simulink model "Single Phase to Ground Fault"  (R2023a)
settings: Solver=ode3  StartTime=0.0  StopTime=1  FixedStep=Ts  RelTol=1e-4  EnableMultiTasking=on
undefined symbols (not defined in the file): Ts
libraries: spsMeanLib x13, spsabctodq0Lib x12, slpidlib x8, spsThreePhaseSeriesRLCBranchLib x7, spsThreePhaseVIMeasurementLib x7, spsSeriesRLCBranchLib x6, spsPower3phInstantaneousLib x5, spspowerguiLib x3, spsPWMGenerator2LevelLib x2, spsdq0toabcLib x2, spsGroundLib x2, spsUniversalBridgeLib x2
(part 1 of 2)
settings Model: Creator=RAVINDRA  LastModifiedBy=LENOVO
settings SolverCC: AlgebraicLoopSolver=TrustRegion
settings DataIOCC: LimitDataPoints=on  SaveFormat=Array  ReturnWorkspaceOutputs=off
settings OptimizationCC: LifeSpan=inf
settings DebuggingCC: SolverPrmCheckMsg=warning  UnconnectedInputMsg=warning  UnconnectedOutputMsg=warning  UnconnectedLineMsg=warning  SFUnexpectedBacktrackingDiag=warning  SFNoUnconditionalDefaultTransitionDiag=warning  SFExecutionAtInitializationDiag=none  ArithmeticOperatorsInVariantConditions=warning
settings HardwareCC: ProdBitPerPointer=32  ProdBitPerSizeT=32  ProdBitPerPtrDiffT=32  ProdLargestAtomicFloat=None  ProdIntDivRoundTo=Undefined  ProdEndianess=Unspecified  ProdWordSize=32  ProdHWDeviceType=32-bit Generic
settings ModelReferenceCC: PropagateSignalLabelsOutOfModel=off
settings SFSimCC: SimUseLocalCustomCode=off  CustomCodeUndefinedFunction=UseInterfaceOnly
settings RTWCC: RTWUseLocalCustomCode=off
settings CodeAppCC: StateflowObjectComments=on
settings GRTTargetCC: TargetLangStandard=C89/C90 (ANSI)
settings ConfigComp: CovMetricSettings=dw  CovSaveCumulativeToWorkspaceVar=on  CovSaveSingleToWorkspaceVar=on  CovExternalEMLEnable=off  CovSFcnEnable=off
settings SimscapeCC: SimscapeNormalizeSystem=off

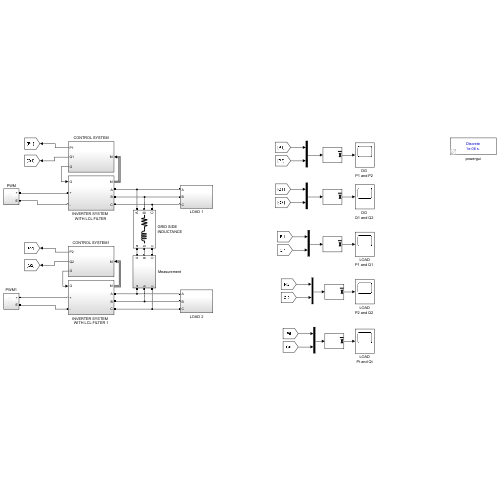
[thumbnail: Simulink's stored preview of the top-level diagram]
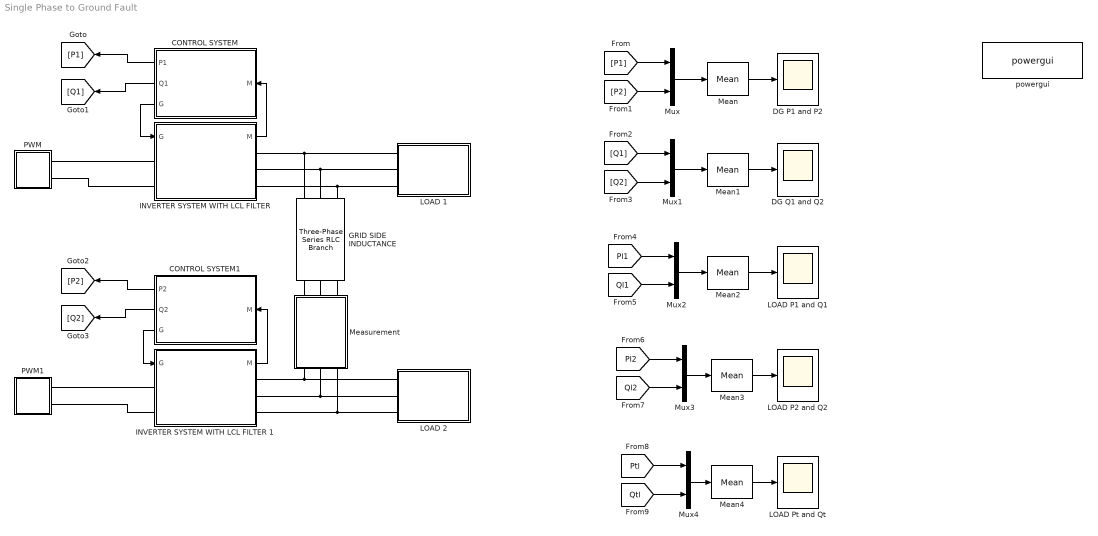
== system Single Phase to Ground Fault ==
  CONTROL SYSTEM : Subsystem
  CONTROL SYSTEM1 : Subsystem
  "DG P1 and P2 " : Scope
  "DG Q1 and Q2 " : Scope
  GRID SIDE INDUCTANCE : spsThreePhaseSeriesRLCBranchLib/Three-Phase Series RLC Branch  LConnTagsString=A|B|C  RConnTagsString=A|B|C  BranchType=RL  Resistance=.55  Inductance=20e-5  Capacitance=1e-6  Measurements=None
  "INVERTER SYSTEM WITH LCL FILTER " : Subsystem
  INVERTER SYSTEM WITH LCL FILTER 1 : Subsystem
  "LOAD P1 and Q1 " : Scope
  "LOAD P2 and Q2 " : Scope
  LOAD Pt and Qt : Scope
  LOAD 1 : Subsystem
  LOAD 2 : Subsystem
  Mean{,1..4} (5 alike) : spsMeanLib/Mean  Freq=60  Vinit=0  Ts=0
  Measurement : Subsystem
  Mux{,1..4} (5 alike) : Mux  Inputs=2
  PWM : Subsystem
  PWM1 : Subsystem
  powergui : spspowerguiLib/powergui  Priority=1  SimulationMode=Discrete  SampleTime=Ts  frequency=60  Iterations=50  frequencyindice=0  Pbase=100e6  ErrMax=1e-4  UnitsV=kV  UnitsW=MW  buscounter=0  FunctionMessages=off  echomessages=off  EnableUseOfTLC=off  CurrentSourceSwitches=off  DisableSnubberDevices=off  DisableRonSwitches=off  DisableVfSwitches=off  DisplayEquations=off  AutomaticDiscreteSolvers=off  SolverType=Tustin  Interpol=off  ExternalGateDelay=off  methode=off  Ts=0  x0status=blocks  SPID=off  SwTol=0  HookPort=off  NonlinearTolerance=1e-4  nMaxIteration=100  ContinueOnMaxIteration=off  RestoreLinks=warning  ResistiveCurrentMeasurement=off  Frange=[0:2:500]  Ylog=off  Xlog=on  ShowGrid=off  save=off  variable=ZData  structure=0  ZoomFFT=off  StartTime=0.0  cycles=1  DisplayStyle=1  fundamental=60  FreqAxis=off  MaxFrequency=1000  frequencyindicesteady=1  RmsSteady=1  display=off
  wires:
  "INVERTER SYSTEM WITH LCL FILTER "/1(M) -> CONTROL SYSTEM/1(M)
  CONTROL SYSTEM/3(G) -> "INVERTER SYSTEM WITH LCL FILTER "/1(G)
  INVERTER SYSTEM WITH LCL FILTER 1/1(M) -> CONTROL SYSTEM1/1(M)
  CONTROL SYSTEM1/3(G) -> INVERTER SYSTEM WITH LCL FILTER 1/1(G)
  CONTROL SYSTEM/1(P1) -> [P1]
  CONTROL SYSTEM/2(Q1) -> [Q1]
  CONTROL SYSTEM1/1(P2) -> [P2]
  CONTROL SYSTEM1/2(Q2) -> [Q2]
  [P1] -> Mux/1
  [P2] -> Mux/2
  Mux/1 -> Mean/1
  [Q1] -> Mux1/1
  [Q2] -> Mux1/2
  [Pl1] -> Mux2/1
  [Ql1] -> Mux2/2
  Mux2/1 -> Mean2/1
  [Pl2] -> Mux3/1
  [Ql2] -> Mux3/2
  [Ptl] -> Mux4/1
  [Qtl] -> Mux4/2
  Mux1/1 -> Mean1/1
  Mux3/1 -> Mean3/1
  Mux4/1 -> Mean4/1
  Mean/1 -> "DG P1 and P2 "/1
  Mean1/1 -> "DG Q1 and Q2 "/1
  Mean2/1 -> "LOAD P1 and Q1 "/1
  Mean3/1 -> "LOAD P2 and Q2 "/1
  Mean4/1 -> LOAD Pt and Qt/1
  connections:
  PWM/LConn1 -- "INVERTER SYSTEM WITH LCL FILTER "/LConn1
  "INVERTER SYSTEM WITH LCL FILTER "/LConn2 -- PWM/LConn2
  LOAD 1/LConn1 -- "INVERTER SYSTEM WITH LCL FILTER "/RConn1 -- GRID SIDE INDUCTANCE/LConn1
  LOAD 1/LConn2 -- "INVERTER SYSTEM WITH LCL FILTER "/RConn2 -- GRID SIDE INDUCTANCE/LConn2
  LOAD 1/LConn3 -- "INVERTER SYSTEM WITH LCL FILTER "/RConn3 -- GRID SIDE INDUCTANCE/LConn3
  INVERTER SYSTEM WITH LCL FILTER 1/RConn1 -- Measurement/LConn1 -- LOAD 2/LConn1
  INVERTER SYSTEM WITH LCL FILTER 1/RConn2 -- Measurement/LConn2 -- LOAD 2/LConn2
  INVERTER SYSTEM WITH LCL FILTER 1/RConn3 -- Measurement/LConn3 -- LOAD 2/LConn3
  INVERTER SYSTEM WITH LCL FILTER 1/LConn1 -- PWM1/LConn1
  PWM1/LConn2 -- INVERTER SYSTEM WITH LCL FILTER 1/LConn2
  Measurement/RConn1 -- GRID SIDE INDUCTANCE/RConn1
  Measurement/RConn2 -- GRID SIDE INDUCTANCE/RConn2
  Measurement/RConn3 -- GRID SIDE INDUCTANCE/RConn3

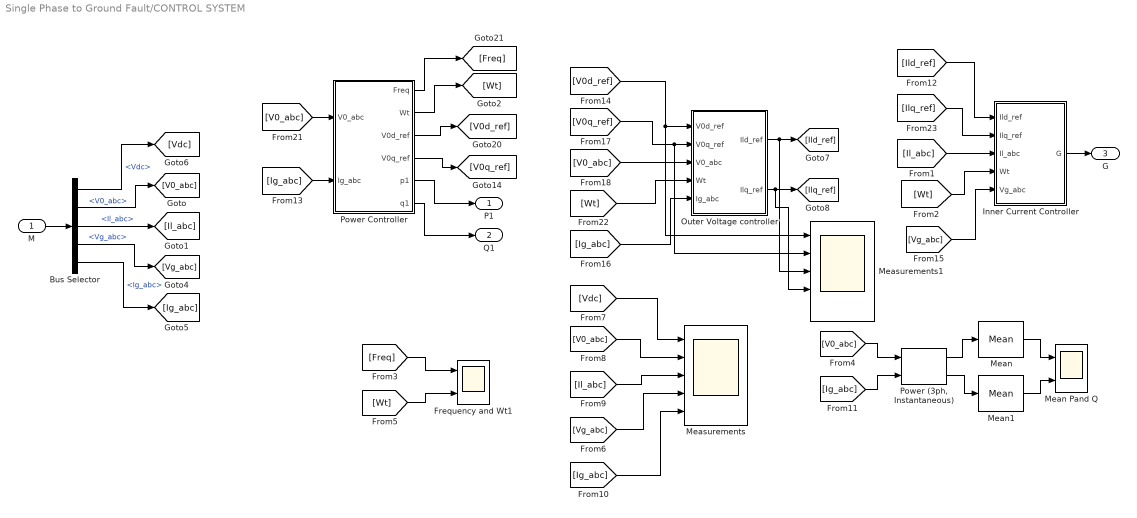
== system Single Phase to Ground Fault/CONTROL SYSTEM ==
  M : Inport
  Bus Selector : BusSelector  OutputSignals=Vdc,V0_abc,Il_abc,Vg_abc,Ig_abc
  Frequency and Wt1 : Scope  NumInputPorts=2
  Inner Current Controller : Subsystem
  Mean : spsMeanLib/Mean  Freq=50  Vinit=0  Ts=0
  Mean Pand Q : Scope  NumInputPorts=2
  Mean1 : spsMeanLib/Mean  Freq=50  Vinit=0  Ts=0
  Measurements : Scope  NumInputPorts=5
  Measurements1 : Scope  NumInputPorts=5
  Outer Voltage controller : Subsystem
  "Power (3ph, Instantaneous)" : spsPower3phInstantaneousLib/Power (3ph, Instantaneous)
  Power Controller : Subsystem
  P1 : Outport
  Q1 : Outport  Port=2
  G : Outport  Port=3
  wires:
  M/1 -> Bus Selector/1
  Bus Selector/1 -> [Vdc]  "<Vdc>"
  Bus Selector/2 -> [V0_abc]  "<V0_abc>"
  Bus Selector/3 -> [Il_abc]  "<Il_abc>"
  Bus Selector/4 -> [Vg_abc]  "<Vg_abc>"
  Bus Selector/5 -> [Ig_abc]  "<Ig_abc>"
  [Vg_abc] -> Measurements/4
  [Vdc] -> Measurements/1
  [V0_abc] -> Measurements/2
  [Il_abc] -> Measurements/3
  [Ig_abc] -> Measurements/5
  [V0_abc] -> Power Controller/1(V0_abc)
  [Ig_abc] -> Power Controller/2(Ig_abc)
  Power Controller/1(Freq) -> [Freq]
  Power Controller/3(V0d_ref) -> [V0d_ref]
  Power Controller/4(V0q_ref) -> [V0q_ref]
  [Wt] -> Frequency and Wt1/2
  Power Controller/2(Wt) -> [Wt]
  [V0d_ref] -> Measurements1/1, Outer Voltage controller/1(V0d_ref)
  [V0q_ref] -> Measurements1/2, Outer Voltage controller/2(V0q_ref)
  [V0_abc] -> Outer Voltage controller/3(V0_abc)
  [Wt] -> Outer Voltage controller/4(Wt)
  Outer Voltage controller/1(Ild_ref) -> Measurements1/3, [Ild_ref]
  Outer Voltage controller/2(Ilq_ref) -> Measurements1/4, [Ilq_ref]
  [Freq] -> Frequency and Wt1/1
  [Ild_ref] -> Inner Current Controller/1(Ild_ref)
  [Ilq_ref] -> Inner Current Controller/2(Ilq_ref)
  [Il_abc] -> Inner Current Controller/3(Il_abc)
  Inner Current Controller/1(G) -> G/1
  [Wt] -> Inner Current Controller/4(Wt)
  [Vg_abc] -> Inner Current Controller/5(Vg_abc)
  [Ig_abc] -> Outer Voltage controller/5(Ig_abc)
  Power Controller/5(p1) -> P1/1
  Power Controller/6(q1) -> Q1/1
  [Ig_abc] -> "Power (3ph, Instantaneous)"/2
  [V0_abc] -> "Power (3ph, Instantaneous)"/1
  "Power (3ph, Instantaneous)"/1 -> Mean/1
  Mean/1 -> Mean Pand Q/1
  Mean1/1 -> Mean Pand Q/2
  "Power (3ph, Instantaneous)"/2 -> Mean1/1

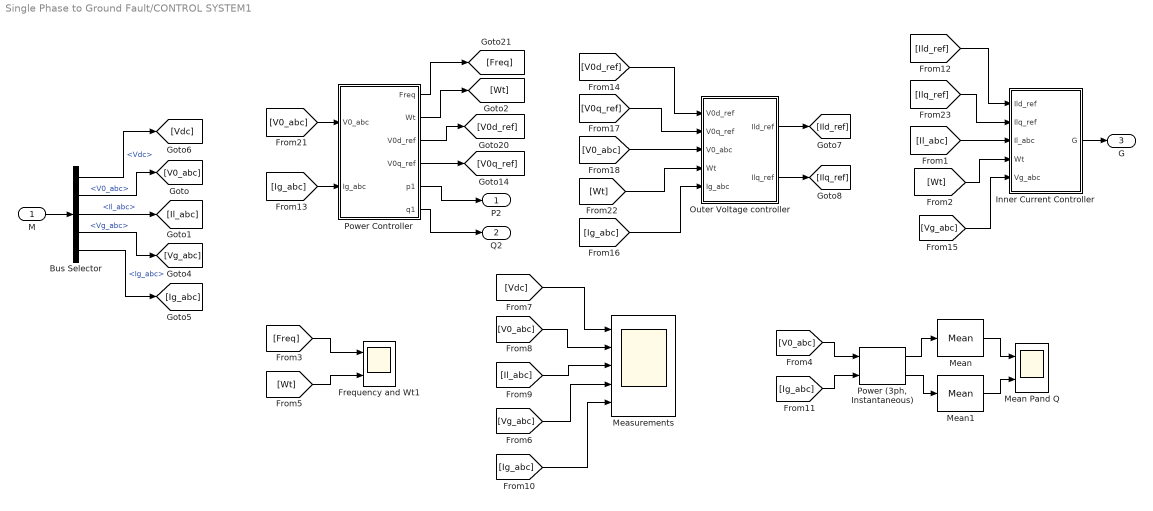
== system Single Phase to Ground Fault/CONTROL SYSTEM1 ==
  M : Inport
  Bus Selector : BusSelector  OutputSignals=Vdc,V0_abc,Il_abc,Vg_abc,Ig_abc
  Frequency and Wt1 : Scope  NumInputPorts=2
  Inner Current Controller : Subsystem
  Mean : spsMeanLib/Mean  Freq=50  Vinit=0  Ts=0
  Mean Pand Q : Scope  NumInputPorts=2
  Mean1 : spsMeanLib/Mean  Freq=50  Vinit=0  Ts=0
  Measurements : Scope  NumInputPorts=5
  Outer Voltage controller : Subsystem
  "Power (3ph, Instantaneous)" : spsPower3phInstantaneousLib/Power (3ph, Instantaneous)
  Power Controller : Subsystem
  P2 : Outport
  Q2 : Outport  Port=2
  G : Outport  Port=3
  wires:
  [Ig_abc] -> Outer Voltage controller/5(Ig_abc)
  [Vg_abc] -> Inner Current Controller/5(Vg_abc)
  [Wt] -> Inner Current Controller/4(Wt)
  Inner Current Controller/1(G) -> G/1
  [Il_abc] -> Inner Current Controller/3(Il_abc)
  [Ilq_ref] -> Inner Current Controller/2(Ilq_ref)
  [Ild_ref] -> Inner Current Controller/1(Ild_ref)
  "Power (3ph, Instantaneous)"/2 -> Mean1/1
  Mean1/1 -> Mean Pand Q/2
  Mean/1 -> Mean Pand Q/1
  "Power (3ph, Instantaneous)"/1 -> Mean/1
  [V0_abc] -> "Power (3ph, Instantaneous)"/1
  [Ig_abc] -> "Power (3ph, Instantaneous)"/2
  [Freq] -> Frequency and Wt1/1
  Outer Voltage controller/2(Ilq_ref) -> [Ilq_ref]
  Outer Voltage controller/1(Ild_ref) -> [Ild_ref]
  [Wt] -> Outer Voltage controller/4(Wt)
  [V0_abc] -> Outer Voltage controller/3(V0_abc)
  [V0q_ref] -> Outer Voltage controller/2(V0q_ref)
  [V0d_ref] -> Outer Voltage controller/1(V0d_ref)
  [Wt] -> Frequency and Wt1/2
  [Ig_abc] -> Measurements/5
  [Il_abc] -> Measurements/3
  [V0_abc] -> Measurements/2
  [Vdc] -> Measurements/1
  [Vg_abc] -> Measurements/4
  Bus Selector/5 -> [Ig_abc]  "<Ig_abc>"
  Bus Selector/4 -> [Vg_abc]  "<Vg_abc>"
  Bus Selector/3 -> [Il_abc]  "<Il_abc>"
  Bus Selector/2 -> [V0_abc]  "<V0_abc>"
  Bus Selector/1 -> [Vdc]  "<Vdc>"
  M/1 -> Bus Selector/1
  [V0_abc] -> Power Controller/1(V0_abc)
  [Ig_abc] -> Power Controller/2(Ig_abc)
  Power Controller/1(Freq) -> [Freq]
  Power Controller/3(V0d_ref) -> [V0d_ref]
  Power Controller/4(V0q_ref) -> [V0q_ref]
  Power Controller/2(Wt) -> [Wt]
  Power Controller/5(p1) -> P2/1
  Power Controller/6(q1) -> Q2/1

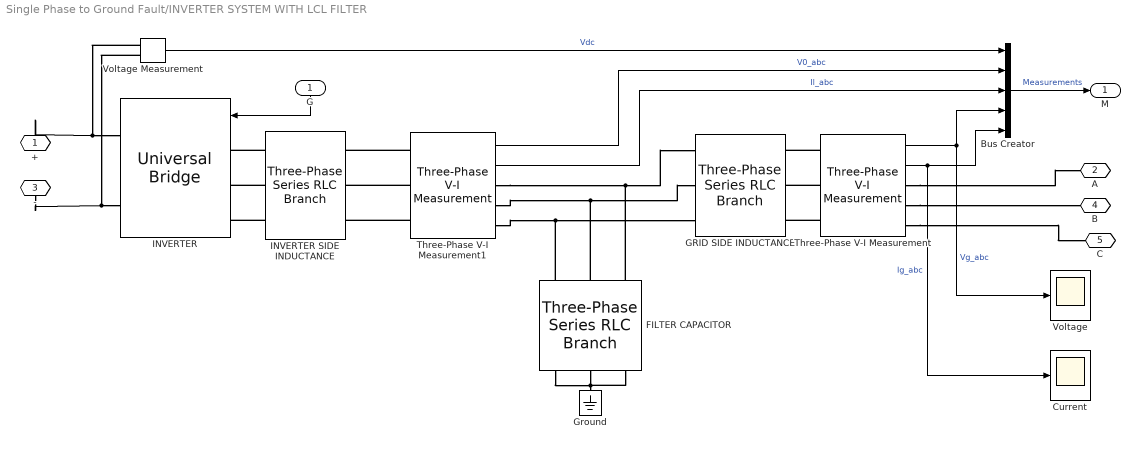
== system Single Phase to Ground Fault/INVERTER SYSTEM WITH LCL FILTER  ==
  G : Inport
  Bus Creator : BusCreator  Inputs=5
  Current : Scope
  FILTER CAPACITOR : spsThreePhaseSeriesRLCBranchLib/Three-Phase Series RLC Branch  LConnTagsString=A|B|C  RConnTagsString=A|B|C  BranchType=RC  Resistance=5  Inductance=1e-3  Capacitance=15e-6  Measurements=None
  GRID SIDE INDUCTANCE : spsThreePhaseSeriesRLCBranchLib/Three-Phase Series RLC Branch  LConnTagsString=A|B|C  RConnTagsString=A|B|C  BranchType=RL  Resistance=0.2  Inductance=1e-3  Capacitance=1e-6  Measurements=None
  Ground : spsGroundLib/Ground  LConnTagsString=a
  INVERTER : spsUniversalBridgeLib/Universal Bridge  Arms=3  SnubberResistance=1e5  SnubberCapacitance=inf  Device=IGBT / Diodes  Ron=1e-3  Lon=0  ForwardVoltages="[  0  0  ]"  ForwardVoltage=0  GTOparameters=[ 10e-6 , 20e-6 ]  IGBTparameters=[ 1e-6 , 2e-6 ]  Measurements=None  Measurements_2=None  converterType=Rectifier
  INVERTER SIDE INDUCTANCE : spsThreePhaseSeriesRLCBranchLib/Three-Phase Series RLC Branch  LConnTagsString=A|B|C  RConnTagsString=A|B|C  BranchType=RL  Resistance=0.2  Inductance=2e-3  Capacitance=1e-6  Measurements=None
  Three-Phase V-I Measurement : spsThreePhaseVIMeasurementLib/Three-Phase V-I Measurement  VoltageMeasurement=phase-to-ground  SetLabelV=off  LabelV=Vabc  Vpu=off  VpuLL=off  CurrentMeasurement=yes  SetLabelI=off  LabelI=Iabc  Ipu=off  Pbase=100e6  Vbase=500e3  OutputType=Complex  PhasorSimulation=off  PSBequivalent=0
  Three-Phase V-I Measurement1 : spsThreePhaseVIMeasurementLib/Three-Phase V-I Measurement  VoltageMeasurement=phase-to-ground  SetLabelV=off  LabelV=V0_abc  Vpu=off  VpuLL=off  CurrentMeasurement=yes  SetLabelI=off  LabelI=Iabc  Ipu=off  Pbase=100e6  Vbase=500e3  OutputType=Complex  PhasorSimulation=off  PSBequivalent=0
  Voltage : Scope
  Voltage Measurement : spsVoltageMeasurementLib/Voltage Measurement  PhasorSimulation=off  OutputType=Complex  PSBequivalent=0
  + : PMIOPort  Side=Left
  A : PMIOPort  Port=2  Side=Right
  - : PMIOPort  Port=3  Side=Left
  B : PMIOPort  Port=4  Side=Right
  C : PMIOPort  Port=5  Side=Right
  M : Outport
  wires:
  Bus Creator/1 -> M/1  "Measurements"
  G/1 -> INVERTER/1
  Three-Phase V-I Measurement/1 -> Voltage/1, Bus Creator/4  "Vg_abc"
  Three-Phase V-I Measurement1/1 -> Bus Creator/2  "V0_abc"
  Three-Phase V-I Measurement1/2 -> Bus Creator/3  "Il_abc"
  Voltage Measurement/1 -> Bus Creator/1  "Vdc"
  Three-Phase V-I Measurement/2 -> Current/1, Bus Creator/5  "Ig_abc"
  connections:
  INVERTER SIDE INDUCTANCE/LConn1 -- INVERTER/LConn1
  Three-Phase V-I Measurement1/LConn1 -- INVERTER SIDE INDUCTANCE/RConn1
  Three-Phase V-I Measurement1/LConn2 -- INVERTER SIDE INDUCTANCE/RConn2
  Voltage Measurement/LConn2 -- -/RConn1 -- INVERTER/RConn2
  Three-Phase V-I Measurement1/LConn3 -- INVERTER SIDE INDUCTANCE/RConn3
  Voltage Measurement/LConn1 -- +/RConn1 -- INVERTER/RConn1
  FILTER CAPACITOR/LConn2 -- GRID SIDE INDUCTANCE/LConn2 -- Three-Phase V-I Measurement1/RConn2
  Three-Phase V-I Measurement/RConn1 -- A/RConn1
  Three-Phase V-I Measurement/RConn3 -- C/RConn1
  INVERTER SIDE INDUCTANCE/LConn3 -- INVERTER/LConn3
  INVERTER SIDE INDUCTANCE/LConn2 -- INVERTER/LConn2
  Three-Phase V-I Measurement/RConn2 -- B/RConn1
  Three-Phase V-I Measurement/LConn1 -- GRID SIDE INDUCTANCE/RConn1
  Three-Phase V-I Measurement/LConn2 -- GRID SIDE INDUCTANCE/RConn2
  FILTER CAPACITOR/LConn1 -- GRID SIDE INDUCTANCE/LConn3 -- Three-Phase V-I Measurement1/RConn3
  FILTER CAPACITOR/RConn1 -- FILTER CAPACITOR/RConn3 -- Ground/LConn1 -- FILTER CAPACITOR/RConn2
  FILTER CAPACITOR/LConn3 -- GRID SIDE INDUCTANCE/LConn1 -- Three-Phase V-I Measurement1/RConn1
  Three-Phase V-I Measurement/LConn3 -- GRID SIDE INDUCTANCE/RConn3

== system Single Phase to Ground Fault/INVERTER SYSTEM WITH LCL FILTER 1 ==
  G : Inport
  Bus Creator : BusCreator  Inputs=5
  FILTER CAPACITOR : spsThreePhaseSeriesRLCBranchLib/Three-Phase Series RLC Branch  LConnTagsString=A|B|C  RConnTagsString=A|B|C  BranchType=RC  Resistance=5  Inductance=1e-3  Capacitance=15e-6  Measurements=None
  GRID SIDE INDUCTANCE : spsThreePhaseSeriesRLCBranchLib/Three-Phase Series RLC Branch  LConnTagsString=A|B|C  RConnTagsString=A|B|C  BranchType=RL  Resistance=0.2  Inductance=1e-3  Capacitance=1e-6  Measurements=None
  Ground : spsGroundLib/Ground  LConnTagsString=a
  INVERTER : spsUniversalBridgeLib/Universal Bridge  Arms=3  SnubberResistance=1e5  SnubberCapacitance=inf  Device=IGBT / Diodes  Ron=1e-3  Lon=0  ForwardVoltages="[  0  0  ]"  ForwardVoltage=0  GTOparameters=[ 10e-6 , 20e-6 ]  IGBTparameters=[ 1e-6 , 2e-6 ]  Measurements=None  Measurements_2=None  converterType=Rectifier
  INVERTER SIDE INDUCTANCE : spsThreePhaseSeriesRLCBranchLib/Three-Phase Series RLC Branch  LConnTagsString=A|B|C  RConnTagsString=A|B|C  BranchType=RL  Resistance=0.2  Inductance=2e-3  Capacitance=1e-6  Measurements=None
  Three-Phase V-I Measurement : spsThreePhaseVIMeasurementLib/Three-Phase V-I Measurement  VoltageMeasurement=phase-to-ground  SetLabelV=off  LabelV=Vabc  Vpu=off  VpuLL=off  CurrentMeasurement=yes  SetLabelI=off  LabelI=Iabc  Ipu=off  Pbase=100e6  Vbase=500e3  OutputType=Complex  PhasorSimulation=off  PSBequivalent=0
  Three-Phase V-I Measurement1 : spsThreePhaseVIMeasurementLib/Three-Phase V-I Measurement  VoltageMeasurement=phase-to-ground  SetLabelV=off  LabelV=V0_abc  Vpu=off  VpuLL=off  CurrentMeasurement=yes  SetLabelI=off  LabelI=Iabc  Ipu=off  Pbase=100e6  Vbase=500e3  OutputType=Complex  PhasorSimulation=off  PSBequivalent=0
  Voltage Measurement : spsVoltageMeasurementLib/Voltage Measurement  PhasorSimulation=off  OutputType=Complex  PSBequivalent=0
  + : PMIOPort  Side=Left
  A : PMIOPort  Port=2  Side=Right
  - : PMIOPort  Port=3  Side=Left
  B : PMIOPort  Port=4  Side=Right
  C : PMIOPort  Port=5  Side=Right
  M : Outport
  wires:
  Three-Phase V-I Measurement/2 -> Bus Creator/5  "Ig_abc"
  Voltage Measurement/1 -> Bus Creator/1  "Vdc"
  Three-Phase V-I Measurement1/2 -> Bus Creator/3  "Il_abc"
  Three-Phase V-I Measurement1/1 -> Bus Creator/2  "V0_abc"
  Three-Phase V-I Measurement/1 -> Bus Creator/4  "Vg_abc"
  G/1 -> INVERTER/1
  Bus Creator/1 -> M/1  "Measurements"
  connections:
  Three-Phase V-I Measurement/LConn3 -- GRID SIDE INDUCTANCE/RConn3
  Three-Phase V-I Measurement1/RConn1 -- GRID SIDE INDUCTANCE/LConn1 -- FILTER CAPACITOR/LConn3
  FILTER CAPACITOR/RConn2 -- Ground/LConn1 -- FILTER CAPACITOR/RConn3 -- FILTER CAPACITOR/RConn1
  Three-Phase V-I Measurement1/RConn3 -- GRID SIDE INDUCTANCE/LConn3 -- FILTER CAPACITOR/LConn1
  Three-Phase V-I Measurement/LConn2 -- GRID SIDE INDUCTANCE/RConn2
  Three-Phase V-I Measurement/LConn1 -- GRID SIDE INDUCTANCE/RConn1
  Three-Phase V-I Measurement/RConn2 -- B/RConn1
  INVERTER SIDE INDUCTANCE/LConn2 -- INVERTER/LConn2
  INVERTER SIDE INDUCTANCE/LConn3 -- INVERTER/LConn3
  Three-Phase V-I Measurement/RConn3 -- C/RConn1
  Three-Phase V-I Measurement/RConn1 -- A/RConn1
  Three-Phase V-I Measurement1/RConn2 -- GRID SIDE INDUCTANCE/LConn2 -- FILTER CAPACITOR/LConn2
  INVERTER/RConn1 -- +/RConn1 -- Voltage Measurement/LConn1
  Three-Phase V-I Measurement1/LConn3 -- INVERTER SIDE INDUCTANCE/RConn3
  INVERTER/RConn2 -- -/RConn1 -- Voltage Measurement/LConn2
  Three-Phase V-I Measurement1/LConn2 -- INVERTER SIDE INDUCTANCE/RConn2
  Three-Phase V-I Measurement1/LConn1 -- INVERTER SIDE INDUCTANCE/RConn1
  INVERTER SIDE INDUCTANCE/LConn1 -- INVERTER/LConn1

== system Single Phase to Ground Fault/LOAD 1 ==
  Mean : spsMeanLib/Mean  Freq=50  Vinit=0  Ts=0
  Mean Pand Q : Scope  NumInputPorts=2
  Mean1 : spsMeanLib/Mean  Freq=50  Vinit=0  Ts=0
  "Power (3ph, Instantaneous)" : spsPower3phInstantaneousLib/Power (3ph, Instantaneous)
  Three-Phase Series RLC Load : spsThreePhaseSeriesRLCLoadLib/Three-Phase Series RLC Load  LConnTagsString=A|B|C  Configuration=Y (grounded)  NominalVoltage=400  Vabc=[1e3 1e3 1e3]  Vabcp=[1e3 1e3 1e3]  NominalFrequency=50  UnbalancedPower=off  ActivePower=7000  InductivePower=0  CapacitivePower=0  Pabc=[10e3 9e3 11e3]  QLabc=[100 90 110]  QCabc=[100 90 110]  Pabcp=[10e3 9e3 11e3]  QLabcp=[100 90 110]  QCabcp=[100 90 110]  Measurements=None  LoadType=constant Z
  Three-Phase V-I Measurement : spsThreePhaseVIMeasurementLib/Three-Phase V-I Measurement  VoltageMeasurement=phase-to-ground  SetLabelV=off  LabelV=Vabc  Vpu=off  VpuLL=off  CurrentMeasurement=yes  SetLabelI=off  LabelI=Iabc  Ipu=off  Pbase=100e6  Vbase=500e3  OutputType=Complex  PhasorSimulation=off  PSBequivalent=0
  Three-Phase Fault : spsThreePhaseFaultLib/Three-Phase Fault  InitialStates=0  FaultA=on  FaultB=off  FaultC=off  GroundFault=on  SwitchTimes=[0.1 0.168]  External=off  SwitchStatus=NaN  FaultResistance=8  GroundResistance=0.01  SnubberResistance=1e6  SnubberCapacitance=inf  Measurements=None
  A : PMIOPort  Side=Left
  B : PMIOPort  Port=2  Side=Left
  C : PMIOPort  Port=3  Side=Left
  tag scope: Pl1=global, Ql1=global
  wires:
  [Il1_abc] -> "Power (3ph, Instantaneous)"/2
  [Vl1_abc] -> "Power (3ph, Instantaneous)"/1
  "Power (3ph, Instantaneous)"/1 -> [Pl1], Mean/1
  Mean/1 -> Mean Pand Q/1
  Mean1/1 -> Mean Pand Q/2
  "Power (3ph, Instantaneous)"/2 -> [Ql1], Mean1/1
  Three-Phase V-I Measurement/2 -> [Il1_abc]
  Three-Phase V-I Measurement/1 -> [Vl1_abc]
  connections:
  Three-Phase V-I Measurement/LConn1 -- Three-Phase Fault/LConn1 -- A/RConn1
  Three-Phase V-I Measurement/LConn2 -- Three-Phase Fault/LConn2 -- B/RConn1
  Three-Phase V-I Measurement/LConn3 -- Three-Phase Fault/LConn3 -- C/RConn1
  Three-Phase V-I Measurement/RConn1 -- Three-Phase Series RLC Load/LConn1
  Three-Phase V-I Measurement/RConn2 -- Three-Phase Series RLC Load/LConn2
  Three-Phase V-I Measurement/RConn3 -- Three-Phase Series RLC Load/LConn3

== system Single Phase to Ground Fault/LOAD 2 ==
  Mean : spsMeanLib/Mean  Freq=50  Vinit=0  Ts=0
  Mean Pand Q : Scope  NumInputPorts=2
  Mean1 : spsMeanLib/Mean  Freq=50  Vinit=0  Ts=0
  "Power (3ph, Instantaneous)" : spsPower3phInstantaneousLib/Power (3ph, Instantaneous)
  Three-Phase Series RLC Load : spsThreePhaseSeriesRLCLoadLib/Three-Phase Series RLC Load  LConnTagsString=A|B|C  Configuration=Y (grounded)  NominalVoltage=400  Vabc=[1e3 1e3 1e3]  Vabcp=[1e3 1e3 1e3]  NominalFrequency=50  UnbalancedPower=off  ActivePower=3000  InductivePower=0  CapacitivePower=0  Pabc=[10e3 9e3 11e3]  QLabc=[100 90 110]  QCabc=[100 90 110]  Pabcp=[10e3 9e3 11e3]  QLabcp=[100 90 110]  QCabcp=[100 90 110]  Measurements=None  LoadType=constant Z
  Three-Phase V-I Measurement : spsThreePhaseVIMeasurementLib/Three-Phase V-I Measurement  VoltageMeasurement=phase-to-ground  SetLabelV=off  LabelV=Vabc  Vpu=off  VpuLL=off  CurrentMeasurement=yes  SetLabelI=off  LabelI=Iabc  Ipu=off  Pbase=100e6  Vbase=500e3  OutputType=Complex  PhasorSimulation=off  PSBequivalent=0
  Three-Phase Fault : spsThreePhaseFaultLib/Three-Phase Fault  InitialStates=0  FaultA=on  FaultB=off  FaultC=off  GroundFault=on  SwitchTimes=[0.1 0.168]  External=off  SwitchStatus=NaN  FaultResistance=8  GroundResistance=0.01  SnubberResistance=1e6  SnubberCapacitance=inf  Measurements=None
  A : PMIOPort  Side=Left
  B : PMIOPort  Port=2  Side=Left
  C : PMIOPort  Port=3  Side=Left
  tag scope: Pl2=global, Ql2=global
  wires:
  [Il2_abc] -> "Power (3ph, Instantaneous)"/2
  [Vl2_abc] -> "Power (3ph, Instantaneous)"/1
  "Power (3ph, Instantaneous)"/1 -> [Pl2], Mean/1
  Mean/1 -> Mean Pand Q/1
  Mean1/1 -> Mean Pand Q/2
  "Power (3ph, Instantaneous)"/2 -> [Ql2], Mean1/1
  Three-Phase V-I Measurement/2 -> [Il2_abc]
  Three-Phase V-I Measurement/1 -> [Vl2_abc]
  connections:
  Three-Phase Series RLC Load/LConn1 -- Three-Phase V-I Measurement/RConn1
  Three-Phase Series RLC Load/LConn3 -- Three-Phase V-I Measurement/RConn3
  Three-Phase Series RLC Load/LConn2 -- Three-Phase V-I Measurement/RConn2
  A/RConn1 -- Three-Phase Fault/LConn1 -- Three-Phase V-I Measurement/LConn1
  B/RConn1 -- Three-Phase Fault/LConn2 -- Three-Phase V-I Measurement/LConn2
  C/RConn1 -- Three-Phase Fault/LConn3 -- Three-Phase V-I Measurement/LConn3

== system Single Phase to Ground Fault/Measurement ==
  "Power (3ph, Instantaneous)" : spsPower3phInstantaneousLib/Power (3ph, Instantaneous)
  Three-Phase V-I Measurement : spsThreePhaseVIMeasurementLib/Three-Phase V-I Measurement  VoltageMeasurement=phase-to-ground  SetLabelV=off  LabelV=Vabc  Vpu=off  VpuLL=off  CurrentMeasurement=yes  SetLabelI=off  LabelI=Iabc  Ipu=off  Pbase=100e6  Vbase=500e3  OutputType=Complex  PhasorSimulation=off  PSBequivalent=0
  A : PMIOPort  Side=Right
  B : PMIOPort  Port=2  Side=Right
  C : PMIOPort  Port=3  Side=Right
  a : PMIOPort  Port=4  Side=Left
  b : PMIOPort  Port=5  Side=Left
  c : PMIOPort  Port=6  Side=Left
  tag scope: Ptl=global, Qtl=global
  wires:
  Three-Phase V-I Measurement/1 -> "Power (3ph, Instantaneous)"/1
  Three-Phase V-I Measurement/2 -> "Power (3ph, Instantaneous)"/2
  "Power (3ph, Instantaneous)"/1 -> [Ptl]
  "Power (3ph, Instantaneous)"/2 -> [Qtl]
  connections:
  A/RConn1 -- Three-Phase V-I Measurement/LConn1
  B/RConn1 -- Three-Phase V-I Measurement/LConn2
  C/RConn1 -- Three-Phase V-I Measurement/LConn3
  a/RConn1 -- Three-Phase V-I Measurement/RConn1
  b/RConn1 -- Three-Phase V-I Measurement/RConn2
  c/RConn1 -- Three-Phase V-I Measurement/RConn3

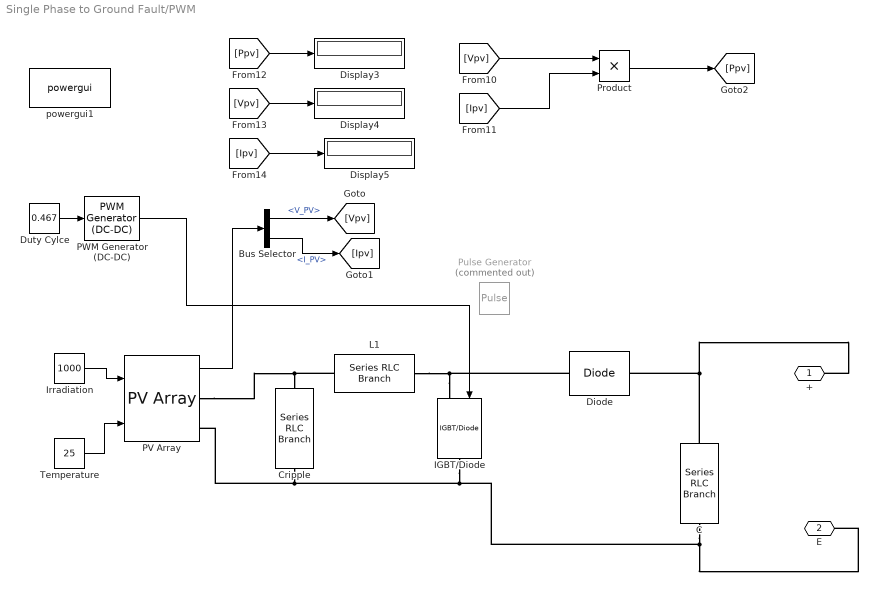
== system Single Phase to Ground Fault/PWM ==
  Bus Selector : BusSelector  OutputSignals=V_PV,I_PV
  C : spsSeriesRLCBranchLib/Series RLC Branch  LConnTagsString=__new0  RConnTagsString=__new0  BranchType=C  Resistance=0  Inductance=0  SetiL0=off  InitialCurrent=0  Capacitance=0.000000207  Setx0=off  InitialVoltage=0  Measurements=None
  Cripple : spsSeriesRLCBranchLib/Series RLC Branch  LConnTagsString=__new0  RConnTagsString=__new0  BranchType=C  Resistance=0  Inductance=0  SetiL0=off  InitialCurrent=0  Capacitance=0.006  Setx0=off  InitialVoltage=0  Measurements=None
  Diode : spsDiodeLib/Diode  Ron=0.001  Lon=0  Vf=0.8  IC=0  UseSnubber=0  Rs=500  Cs=250e-9  Measurements=off
  Display3 : Display
  Display4 : Display
  Display5 : Display
  Duty Cylce : Constant  Value=0.467
  IGBT/Diode : spsIGBTDiodeLib/IGBT//Diode  Ron=1e-3  Rs=1e5  Cs=inf  Measurements=off
  Irradiation : Constant  Value=1000
  L1 : spsSeriesRLCBranchLib/Series RLC Branch  LConnTagsString=__new0  RConnTagsString=__new0  BranchType=L  Resistance=0  Inductance=0.000349  SetiL0=off  InitialCurrent=0  Capacitance=0.006  Setx0=off  InitialVoltage=0  Measurements=None
  PV Array : spsPVArrayLib/PV Array  Npar=5  Nser=10  PlotType=array @ 1000 W/m2 & specified temperatures  S_vec="[ 1000  500  100 ]"  Temp_C_vec="[ 45 25  ]"  ModuleName=User-defined  PlotWhenSelected=off  Pm=200  Ncell=5.8  Voc=41  Isc=6  Vm=40  Im=5  beta_Voc_pc=-0.36099  alpha_Isc_pc=0.102  beta_Voc=-0.14801  alpha_Isc=0.00612  IL=7.0494  I0=8.7017e-23  nI=5.8087  Rsh=8.8608  Rs=0.0024678  RobustModel=off  RobustCellTemperature=25  BAL=on  Tc=1e-6  Tfilter=5e-5
  PWM Generator (DC-DC) : spsPWMGeneratorDCDCLib/PWM Generator (DC-DC)  Fsw=20000  Ts=Ts
  Product : Product
  Pulse Generator : DiscretePulseGenerator  Commented=on  PulseType=Time based  Period=5e-05  PulseWidth=0.002
  Temperature : Constant  Value=25
  powergui1 : spspowerguiLib/powergui  Priority=1  SimulationMode=Discrete  SampleTime=1e-6  frequency=60  Iterations=50  frequencyindice=0  Pbase=100e6  ErrMax=1e-4  UnitsV=kV  UnitsW=MW  buscounter=0  FunctionMessages=off  echomessages=off  EnableUseOfTLC=off  CurrentSourceSwitches=off  DisableSnubberDevices=off  DisableRonSwitches=off  DisableVfSwitches=off  DisplayEquations=off  AutomaticDiscreteSolvers=off  SolverType=Tustin/Backward Euler (TBE)  Interpol=off  ExternalGateDelay=off  methode=off  Ts=100  x0status=blocks  SPID=on  SwTol=0  HookPort=off  NonlinearTolerance=1e-4  nMaxIteration=100  ContinueOnMaxIteration=off  RestoreLinks=warning  ResistiveCurrentMeasurement=off  Frange=[0:2:500]  Ylog=off  Xlog=on  ShowGrid=off  save=off  variable=ZData  structure=0  ZoomFFT=off  StartTime=0.0  cycles=1  DisplayStyle=1  fundamental=60  FreqAxis=off  MaxFrequency=1000  frequencyindicesteady=1  RmsSteady=1  display=off
  + : PMIOPort  Side=Left
  E : PMIOPort  Port=2  Side=Left
  wires:
  [Vpv] -> Display4/1
  Bus Selector/2 -> [Ipv]  "<I_PV>"
  Bus Selector/1 -> [Vpv]  "<V_PV>"
  [Ipv] -> Display5/1
  [Ppv] -> Display3/1
  [Vpv] -> Product/1
  Irradiation/1 -> PV Array/1
  PWM Generator (DC-DC)/1 -> IGBT/Diode/1
  [Ipv] -> Product/2
  Duty Cylce/1 -> PWM Generator (DC-DC)/1
  Product/1 -> [Ppv]
  PV Array/1 -> Bus Selector/1
  Temperature/1 -> PV Array/2
  connections:
  Cripple/LConn1 -- PV Array/RConn1 -- L1/RConn1
  C/LConn1 -- Diode/RConn1 -- +/RConn1
  IGBT/Diode/LConn1 -- L1/LConn1 -- Diode/LConn1
  PV Array/RConn2 -- Cripple/RConn1 -- IGBT/Diode/RConn1 -- C/RConn1 -- E/RConn1

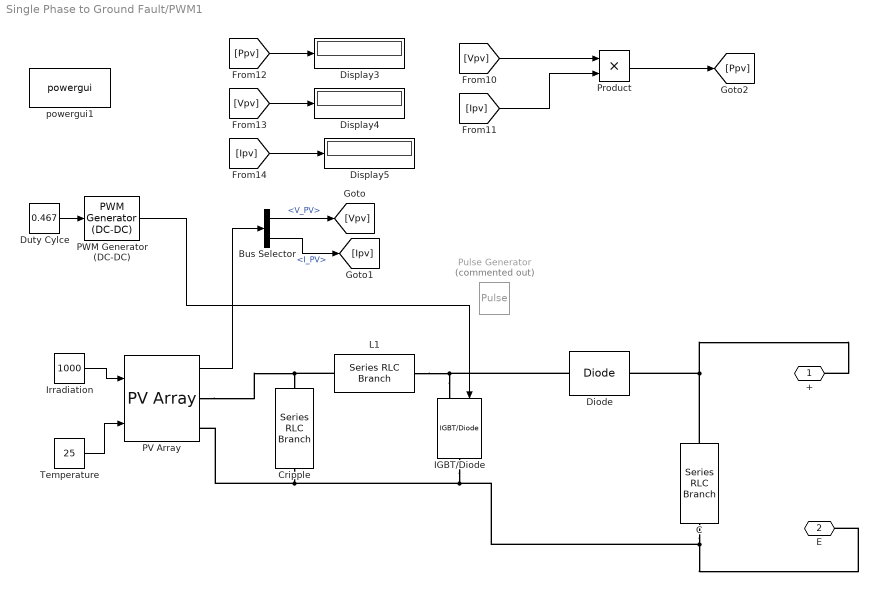
== system Single Phase to Ground Fault/PWM1 ==
  Bus Selector : BusSelector  OutputSignals=V_PV,I_PV
  C : spsSeriesRLCBranchLib/Series RLC Branch  LConnTagsString=__new0  RConnTagsString=__new0  BranchType=C  Resistance=0  Inductance=0  SetiL0=off  InitialCurrent=0  Capacitance=0.000000207  Setx0=off  InitialVoltage=0  Measurements=None
  Cripple : spsSeriesRLCBranchLib/Series RLC Branch  LConnTagsString=__new0  RConnTagsString=__new0  BranchType=C  Resistance=0  Inductance=0  SetiL0=off  InitialCurrent=0  Capacitance=0.006  Setx0=off  InitialVoltage=0  Measurements=None
  Diode : spsDiodeLib/Diode  Ron=0.001  Lon=0  Vf=0.8  IC=0  UseSnubber=0  Rs=500  Cs=250e-9  Measurements=off
  Display3 : Display
  Display4 : Display
  Display5 : Display
  Duty Cylce : Constant  Value=0.467
  IGBT/Diode : spsIGBTDiodeLib/IGBT//Diode  Ron=1e-3  Rs=1e5  Cs=inf  Measurements=off
  Irradiation : Constant  Value=1000
  L1 : spsSeriesRLCBranchLib/Series RLC Branch  LConnTagsString=__new0  RConnTagsString=__new0  BranchType=L  Resistance=0  Inductance=0.000349  SetiL0=off  InitialCurrent=0  Capacitance=0.006  Setx0=off  InitialVoltage=0  Measurements=None
  PV Array : spsPVArrayLib/PV Array  Npar=5  Nser=10  PlotType=array @ 1000 W/m2 & specified temperatures  S_vec="[ 1000  500  100 ]"  Temp_C_vec="[ 45 25  ]"  ModuleName=User-defined  PlotWhenSelected=off  Pm=200  Ncell=5.8  Voc=41  Isc=6  Vm=40  Im=5  beta_Voc_pc=-0.36099  alpha_Isc_pc=0.102  beta_Voc=-0.14801  alpha_Isc=0.00612  IL=7.0494  I0=8.7017e-23  nI=5.8087  Rsh=8.8608  Rs=0.0024678  RobustModel=off  RobustCellTemperature=25  BAL=on  Tc=1e-6  Tfilter=5e-5
  PWM Generator (DC-DC) : spsPWMGeneratorDCDCLib/PWM Generator (DC-DC)  Fsw=20000  Ts=Ts
  Product : Product
  Pulse Generator : DiscretePulseGenerator  Commented=on  PulseType=Time based  Period=5e-05  PulseWidth=0.002
  Temperature : Constant  Value=25
  powergui1 : spspowerguiLib/powergui  Priority=1  SimulationMode=Discrete  SampleTime=1e-6  frequency=60  Iterations=50  frequencyindice=0  Pbase=100e6  ErrMax=1e-4  UnitsV=kV  UnitsW=MW  buscounter=0  FunctionMessages=off  echomessages=off  EnableUseOfTLC=off  CurrentSourceSwitches=off  DisableSnubberDevices=off  DisableRonSwitches=off  DisableVfSwitches=off  DisplayEquations=off  AutomaticDiscreteSolvers=off  SolverType=Tustin/Backward Euler (TBE)  Interpol=off  ExternalGateDelay=off  methode=off  Ts=100  x0status=blocks  SPID=on  SwTol=0  HookPort=off  NonlinearTolerance=1e-4  nMaxIteration=100  ContinueOnMaxIteration=off  RestoreLinks=warning  ResistiveCurrentMeasurement=off  Frange=[0:2:500]  Ylog=off  Xlog=on  ShowGrid=off  save=off  variable=ZData  structure=0  ZoomFFT=off  StartTime=0.0  cycles=1  DisplayStyle=1  fundamental=60  FreqAxis=off  MaxFrequency=1000  frequencyindicesteady=1  RmsSteady=1  display=off
  + : PMIOPort  Side=Left
  E : PMIOPort  Port=2  Side=Left
  wires:
  [Vpv] -> Display4/1
  Bus Selector/2 -> [Ipv]  "<I_PV>"
  Bus Selector/1 -> [Vpv]  "<V_PV>"
  [Ipv] -> Display5/1
  [Ppv] -> Display3/1
  [Vpv] -> Product/1
  Irradiation/1 -> PV Array/1
  PWM Generator (DC-DC)/1 -> IGBT/Diode/1
  [Ipv] -> Product/2
  Duty Cylce/1 -> PWM Generator (DC-DC)/1
  Product/1 -> [Ppv]
  PV Array/1 -> Bus Selector/1
  Temperature/1 -> PV Array/2
  connections:
  Cripple/LConn1 -- PV Array/RConn1 -- L1/RConn1
  C/LConn1 -- Diode/RConn1 -- +/RConn1
  IGBT/Diode/LConn1 -- L1/LConn1 -- Diode/LConn1
  PV Array/RConn2 -- Cripple/RConn1 -- IGBT/Diode/RConn1 -- C/RConn1 -- E/RConn1

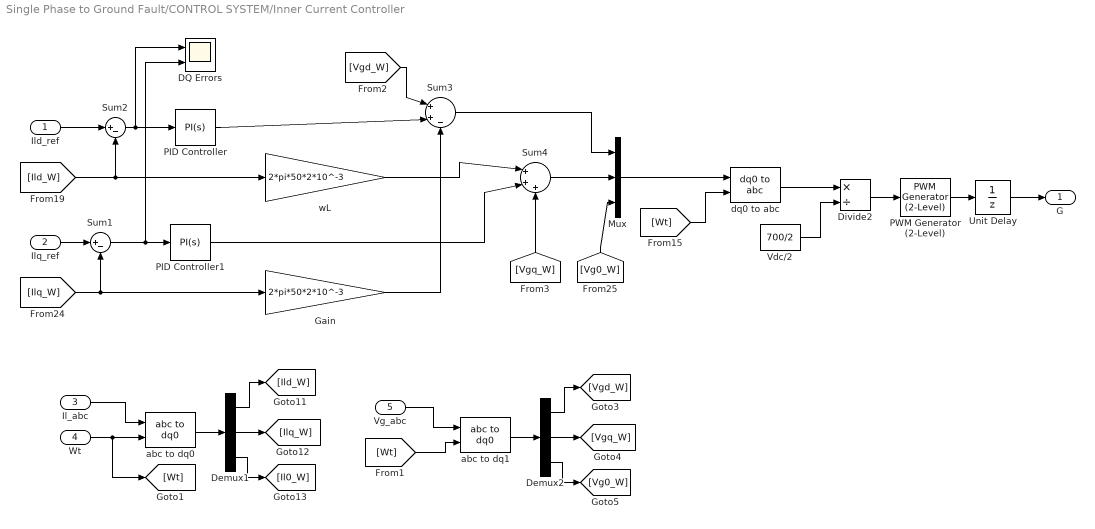
== system Single Phase to Ground Fault/CONTROL SYSTEM/Inner Current Controller ==
  Ild_ref : Inport
  Ilq_ref : Inport  Port=2
  Il_abc : Inport  Port=3
  Wt : Inport  Port=4
  Vg_abc : Inport  Port=5
  DQ Errors : Scope  NumInputPorts=2
  Demux1 : Demux  Outputs=3
  Demux2 : Demux  Outputs=3
  Divide2 : Product  Inputs=*/
  Gain : Gain  Gain=2*pi*50*2*10^-3
  Mux : Mux  Inputs=3
  PID Controller : slpidlib/PID Controller  Controller=PI  Form=Parallel  TimeDomain=Continuous-time  UseExternalTs=off  SampleTime=1  IntegratorMethod=Forward Euler  FilterMethod=Forward Euler  ControllerParametersSource=internal  P=20  I=400  UseKiTs=off  D=0  N=100  UseFilter=on  TunerSelectOption=Transfer Function Based (PID Tuner App)  InitialConditionSource=internal  InitialConditionForIntegrator=0  InitialConditionForFilter=0  DifferentiatorICPrevScaledInput=0  ExternalReset=none  TrackingMode=off  Kt=1  LimitOutput=off  SatLimitsSource=internal  UpperSaturationLimit=inf  LowerSaturationLimit=-inf  LinearizeAsGain=on  AntiWindupMode=none  Kb=1  LimitIntegrator=off  UpperIntegratorSaturationLimit=inf  LowerIntegratorSaturationLimit=-inf  POutMin=[]  POutMax=[]  IOutMin=[]  IOutMax=[]  DOutMin=[]  DOutMax=[]  NOutMin=[]  NOutMax=[]  SumOutMin=[]  SumOutMax=[]  SaturationOutMin=[]  SaturationOutMax=[]  PParamMin=[]  PParamMax=[]  IParamMin=[]  IParamMax=[]  DParamMin=[]  DParamMax=[]  NParamMin=[]  NParamMax=[]  KbParamMin=[]  KbParamMax=[]  KtParamMin=[]  KtParamMax=[]  KbOutMin=[]  KbOutMax=[]  KtOutMin=[]  KtOutMax=[]  IntegratorOutMin=[]  IntegratorOutMax=[]  FilterOutMin=[]  FilterOutMax=[]  SumI1OutMin=[]  SumI1OutMax=[]  SumI2OutMin=[]  SumI2OutMax=[]  SumI3OutMin=[]  SumI3OutMax=[]  SumI4OutMin=[]  SumI4OutMax=[]  SumDOutMin=[]  SumDOutMax=[]  DifferentiatorOutMin=[]  DifferentiatorOutMax=[]  FilterDiffOutCoefMin=[]  FilterDiffOutCoefMax=[]  ReciprocalOutMin=[]  ReciprocalOutMax=[]  SumDenOutMin=[]  SumDenOutMax=[]  SumNumOutMin=[]  SumNumOutMax=[]  DivideOutMin=[]  DivideOutMax=[]  UdiffTsProdOutMin=[]  UdiffTsProdOutMax=[]  NTsProdOutMin=[]  NTsProdOutMax=[]  UintegralTsProdOutMin=[]  UintegralTsProdOutMax=[]  UngainTsProdOutMin=[]  UngainTsProdOutMax=[]  ClampingZeroOutDataTypeStr=Inherit: Inherit via back propagation  ClampingZeroOutMin=[]  ClampingZeroOutMax=[]  FilterDenConstantOutDataTypeStr=Inherit: Inherit via back propagation  FilterDenConstantOutMin=[]  FilterDenConstantOutMax=[]  PCopyOutDataTypeStr=Inherit: Inherit via back propagation  PCopyOutMin=[]  PCopyOutMax=[]  NCopyOutDataTypeStr=Inherit: Inherit via back propagation  NCopyOutMin=[]  NCopyOutMax=[]  IntegratorContinuousStateAttributes=''  IntegratorStateMustResolveToSignalObject=off  IntegratorRTWStateStorageClass=Auto  FilterContinuousStateAttributes=''  FilterStateMustResolveToSignalObject=off  FilterRTWStateStorageClass=Auto  ParallelPVariant=InternalParameters  IdealPVariant=Disabled  IVariant=InternalParameters  DVariant=Disabled  IntegratorVariant=Continuous  SatVariant=Disabled  AWVariant=Passthrough  PCopyVariant=Disabled  TRVariant=Disabled  FdbkBlocksVariant=Forward  IdealPFdbkVariant=Disabled  SatFdbkVariant=Disabled  DerivativeFilterVariant=Disabled  NVariant=Disabled  NCopyVariant=Disabled_SignalSpec  FilterICVariant=Disabled  IntegratorICVariant=InternalICs  ExternalResetVariant=Disabled  TRSumVariant=Passthrough  SumFdbkVariant=Disabled  SumVariant=Sum_PI  TsampFilterVariant=InternalTs  TsampNgainVariant=Passthrough  TsampIntegralVariant=Disabled_SignalSpec  ExternalSaturationOutDataTypeStr=Inherit: Same as second input
  PID Controller1 : slpidlib/PID Controller  Controller=PI  Form=Parallel  TimeDomain=Continuous-time  UseExternalTs=off  SampleTime=1  IntegratorMethod=Forward Euler  FilterMethod=Forward Euler  ControllerParametersSource=internal  P=20  I=400  UseKiTs=off  D=0  N=100  UseFilter=on  TunerSelectOption=Transfer Function Based (PID Tuner App)  InitialConditionSource=internal  InitialConditionForIntegrator=0  InitialConditionForFilter=0  DifferentiatorICPrevScaledInput=0  ExternalReset=none  TrackingMode=off  Kt=1  LimitOutput=off  SatLimitsSource=internal  UpperSaturationLimit=inf  LowerSaturationLimit=-inf  LinearizeAsGain=on  AntiWindupMode=none  Kb=1  LimitIntegrator=off  UpperIntegratorSaturationLimit=inf  LowerIntegratorSaturationLimit=-inf  POutMin=[]  POutMax=[]  IOutMin=[]  IOutMax=[]  DOutMin=[]  DOutMax=[]  NOutMin=[]  NOutMax=[]  SumOutMin=[]  SumOutMax=[]  SaturationOutMin=[]  SaturationOutMax=[]  PParamMin=[]  PParamMax=[]  IParamMin=[]  IParamMax=[]  DParamMin=[]  DParamMax=[]  NParamMin=[]  NParamMax=[]  KbParamMin=[]  KbParamMax=[]  KtParamMin=[]  KtParamMax=[]  KbOutMin=[]  KbOutMax=[]  KtOutMin=[]  KtOutMax=[]  IntegratorOutMin=[]  IntegratorOutMax=[]  FilterOutMin=[]  FilterOutMax=[]  SumI1OutMin=[]  SumI1OutMax=[]  SumI2OutMin=[]  SumI2OutMax=[]  SumI3OutMin=[]  SumI3OutMax=[]  SumI4OutMin=[]  SumI4OutMax=[]  SumDOutMin=[]  SumDOutMax=[]  DifferentiatorOutMin=[]  DifferentiatorOutMax=[]  FilterDiffOutCoefMin=[]  FilterDiffOutCoefMax=[]  ReciprocalOutMin=[]  ReciprocalOutMax=[]  SumDenOutMin=[]  SumDenOutMax=[]  SumNumOutMin=[]  SumNumOutMax=[]  DivideOutMin=[]  DivideOutMax=[]  UdiffTsProdOutMin=[]  UdiffTsProdOutMax=[]  NTsProdOutMin=[]  NTsProdOutMax=[]  UintegralTsProdOutMin=[]  UintegralTsProdOutMax=[]  UngainTsProdOutMin=[]  UngainTsProdOutMax=[]  ClampingZeroOutDataTypeStr=Inherit: Inherit via back propagation  ClampingZeroOutMin=[]  ClampingZeroOutMax=[]  FilterDenConstantOutDataTypeStr=Inherit: Inherit via back propagation  FilterDenConstantOutMin=[]  FilterDenConstantOutMax=[]  PCopyOutDataTypeStr=Inherit: Inherit via back propagation  PCopyOutMin=[]  PCopyOutMax=[]  NCopyOutDataTypeStr=Inherit: Inherit via back propagation  NCopyOutMin=[]  NCopyOutMax=[]  IntegratorContinuousStateAttributes=''  IntegratorStateMustResolveToSignalObject=off  IntegratorRTWStateStorageClass=Auto  FilterContinuousStateAttributes=''  FilterStateMustResolveToSignalObject=off  FilterRTWStateStorageClass=Auto  ParallelPVariant=InternalParameters  IdealPVariant=Disabled  IVariant=InternalParameters  DVariant=Disabled  IntegratorVariant=Continuous  SatVariant=Disabled  AWVariant=Passthrough  PCopyVariant=Disabled  TRVariant=Disabled  FdbkBlocksVariant=Forward  IdealPFdbkVariant=Disabled  SatFdbkVariant=Disabled  DerivativeFilterVariant=Disabled  NVariant=Disabled  NCopyVariant=Disabled_SignalSpec  FilterICVariant=Disabled  IntegratorICVariant=InternalICs  ExternalResetVariant=Disabled  TRSumVariant=Passthrough  SumFdbkVariant=Disabled  SumVariant=Sum_PI  TsampFilterVariant=InternalTs  TsampNgainVariant=Passthrough  TsampIntegralVariant=Disabled_SignalSpec  ExternalSaturationOutDataTypeStr=Inherit: Same as second input
  PWM Generator (2-Level) : spsPWMGenerator2LevelLib/PWM Generator (2-Level)  ModulatorType=Three-phase bridge (6 pulses)  ModulatorMode=Unsynchronized  Fc=15000  Pc=90  nF=27  MinMax="[ -1  1 ]"  SamplingTechnique=Natural  ModulatingSignals=off  m=0.8  Freq=60  Phase=0  Ts=Ts  ShowCarrierOutport=off
  Sum1 : Sum  Inputs=|+-
  Sum2 : Sum  Inputs=|+-
  Sum3 : Sum  Inputs=|++-
  Sum4 : Sum  Inputs=|+++
  Unit Delay : UnitDelay  SampleTime=-1  HasFrameUpgradeWarning=on
  Vdc/2 : Constant  Value=700/2  SampleTime=Ts
  abc to dq0 : spsabctodq0Lib/abc to dq0  Alignment=90 degrees behind phase A axis
  abc to dq1 : spsabctodq0Lib/abc to dq0  Alignment=90 degrees behind phase A axis
  dq0 to abc : spsdq0toabcLib/dq0 to abc  Alignment=90 degrees behind phase A axis
  wL : Gain  Gain=2*pi*50*2*10^-3
  G : Outport
  wires:
  abc to dq0/1 -> Demux1/1
  Demux1/3 -> [Il0_W]
  Mux/1 -> dq0 to abc/1
  Demux1/2 -> [Ilq_W]
  Demux1/1 -> [Ild_W]
  PWM Generator (2-Level)/1 -> Unit Delay/1
  Il_abc/1 -> abc to dq0/1
  Unit Delay/1 -> G/1
  Ilq_ref/1 -> Sum1/1
  Ild_ref/1 -> Sum2/1
  Sum1/1 -> DQ Errors/2, PID Controller1/1
  Sum2/1 -> PID Controller/1, DQ Errors/1
  [Vg0_W] -> Mux/3
  dq0 to abc/1 -> Divide2/1
  Divide2/1 -> PWM Generator (2-Level)/1
  Vdc/2/1 -> Divide2/2
  [Wt] -> dq0 to abc/2
  [Ild_W] -> wL/1, Sum2/2
  [Ilq_W] -> Gain/1, Sum1/2
  PID Controller1/1 -> Sum4/2
  wL/1 -> Sum4/1
  Gain/1 -> Sum3/3
  PID Controller/1 -> Sum3/2
  Sum4/1 -> Mux/2
  Sum3/1 -> Mux/1
  abc to dq1/1 -> Demux2/1
  Demux2/3 -> [Vg0_W]
  Demux2/2 -> [Vgq_W]
  Demux2/1 -> [Vgd_W]
  Vg_abc/1 -> abc to dq1/1
  Wt/1 -> [Wt], abc to dq0/2
  [Wt] -> abc to dq1/2
  [Vgd_W] -> Sum3/1
  [Vgq_W] -> Sum4/3

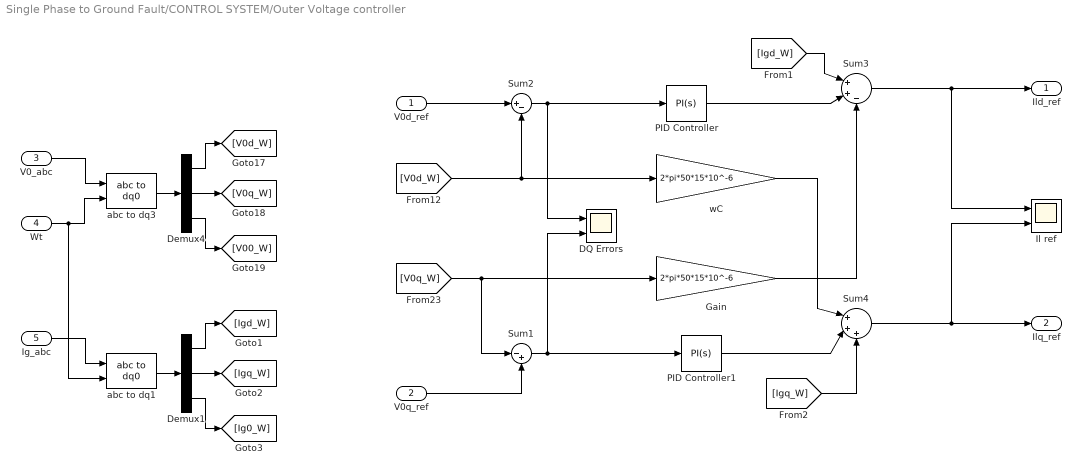
== system Single Phase to Ground Fault/CONTROL SYSTEM/Outer Voltage controller ==
  V0d_ref : Inport
  V0q_ref : Inport  Port=2
  V0_abc : Inport  Port=3
  Wt : Inport  Port=4
  Ig_abc : Inport  Port=5
  DQ Errors : Scope  NumInputPorts=2
  Demux1 : Demux  Outputs=3
  Demux4 : Demux  Outputs=3
  Gain : Gain  Gain=2*pi*50*15*10^-6
  Il ref : Scope  NumInputPorts=2
  PID Controller : slpidlib/PID Controller  Controller=PI  Form=Parallel  TimeDomain=Continuous-time  UseExternalTs=off  SampleTime=1  IntegratorMethod=Forward Euler  FilterMethod=Forward Euler  ControllerParametersSource=internal  P=2  I=10  UseKiTs=off  D=0  N=100  UseFilter=on  TunerSelectOption=Transfer Function Based (PID Tuner App)  InitialConditionSource=internal  InitialConditionForIntegrator=0  InitialConditionForFilter=0  DifferentiatorICPrevScaledInput=0  ExternalReset=none  TrackingMode=off  Kt=1  LimitOutput=off  SatLimitsSource=internal  UpperSaturationLimit=inf  LowerSaturationLimit=-inf  LinearizeAsGain=on  AntiWindupMode=none  Kb=1  LimitIntegrator=off  UpperIntegratorSaturationLimit=inf  LowerIntegratorSaturationLimit=-inf  POutMin=[]  POutMax=[]  IOutMin=[]  IOutMax=[]  DOutMin=[]  DOutMax=[]  NOutMin=[]  NOutMax=[]  SumOutMin=[]  SumOutMax=[]  SaturationOutMin=[]  SaturationOutMax=[]  PParamMin=[]  PParamMax=[]  IParamMin=[]  IParamMax=[]  DParamMin=[]  DParamMax=[]  NParamMin=[]  NParamMax=[]  KbParamMin=[]  KbParamMax=[]  KtParamMin=[]  KtParamMax=[]  KbOutMin=[]  KbOutMax=[]  KtOutMin=[]  KtOutMax=[]  IntegratorOutMin=[]  IntegratorOutMax=[]  FilterOutMin=[]  FilterOutMax=[]  SumI1OutMin=[]  SumI1OutMax=[]  SumI2OutMin=[]  SumI2OutMax=[]  SumI3OutMin=[]  SumI3OutMax=[]  SumI4OutMin=[]  SumI4OutMax=[]  SumDOutMin=[]  SumDOutMax=[]  DifferentiatorOutMin=[]  DifferentiatorOutMax=[]  FilterDiffOutCoefMin=[]  FilterDiffOutCoefMax=[]  ReciprocalOutMin=[]  ReciprocalOutMax=[]  SumDenOutMin=[]  SumDenOutMax=[]  SumNumOutMin=[]  SumNumOutMax=[]  DivideOutMin=[]  DivideOutMax=[]  UdiffTsProdOutMin=[]  UdiffTsProdOutMax=[]  NTsProdOutMin=[]  NTsProdOutMax=[]  UintegralTsProdOutMin=[]  UintegralTsProdOutMax=[]  UngainTsProdOutMin=[]  UngainTsProdOutMax=[]  ClampingZeroOutDataTypeStr=Inherit: Inherit via back propagation  ClampingZeroOutMin=[]  ClampingZeroOutMax=[]  FilterDenConstantOutDataTypeStr=Inherit: Inherit via back propagation  FilterDenConstantOutMin=[]  FilterDenConstantOutMax=[]  PCopyOutDataTypeStr=Inherit: Inherit via back propagation  PCopyOutMin=[]  PCopyOutMax=[]  NCopyOutDataTypeStr=Inherit: Inherit via back propagation  NCopyOutMin=[]  NCopyOutMax=[]  IntegratorContinuousStateAttributes=''  IntegratorStateMustResolveToSignalObject=off  IntegratorRTWStateStorageClass=Auto  FilterContinuousStateAttributes=''  FilterStateMustResolveToSignalObject=off  FilterRTWStateStorageClass=Auto  ParallelPVariant=InternalParameters  IdealPVariant=Disabled  IVariant=InternalParameters  DVariant=Disabled  IntegratorVariant=Continuous  SatVariant=Disabled  AWVariant=Passthrough  PCopyVariant=Disabled  TRVariant=Disabled  FdbkBlocksVariant=Forward  IdealPFdbkVariant=Disabled  SatFdbkVariant=Disabled  DerivativeFilterVariant=Disabled  NVariant=Disabled  NCopyVariant=Disabled_SignalSpec  FilterICVariant=Disabled  IntegratorICVariant=InternalICs  ExternalResetVariant=Disabled  TRSumVariant=Passthrough  SumFdbkVariant=Disabled  SumVariant=Sum_PI  TsampFilterVariant=InternalTs  TsampNgainVariant=Passthrough  TsampIntegralVariant=Disabled_SignalSpec  ExternalSaturationOutDataTypeStr=Inherit: Same as second input
  PID Controller1 : slpidlib/PID Controller  Controller=PI  Form=Parallel  TimeDomain=Continuous-time  UseExternalTs=off  SampleTime=1  IntegratorMethod=Forward Euler  FilterMethod=Forward Euler  ControllerParametersSource=internal  P=2  I=10  UseKiTs=off  D=0  N=100  UseFilter=on  TunerSelectOption=Transfer Function Based (PID Tuner App)  InitialConditionSource=internal  InitialConditionForIntegrator=0  InitialConditionForFilter=0  DifferentiatorICPrevScaledInput=0  ExternalReset=none  TrackingMode=off  Kt=1  LimitOutput=off  SatLimitsSource=internal  UpperSaturationLimit=inf  LowerSaturationLimit=-inf  LinearizeAsGain=on  AntiWindupMode=none  Kb=1  LimitIntegrator=off  UpperIntegratorSaturationLimit=inf  LowerIntegratorSaturationLimit=-inf  POutMin=[]  POutMax=[]  IOutMin=[]  IOutMax=[]  DOutMin=[]  DOutMax=[]  NOutMin=[]  NOutMax=[]  SumOutMin=[]  SumOutMax=[]  SaturationOutMin=[]  SaturationOutMax=[]  PParamMin=[]  PParamMax=[]  IParamMin=[]  IParamMax=[]  DParamMin=[]  DParamMax=[]  NParamMin=[]  NParamMax=[]  KbParamMin=[]  KbParamMax=[]  KtParamMin=[]  KtParamMax=[]  KbOutMin=[]  KbOutMax=[]  KtOutMin=[]  KtOutMax=[]  IntegratorOutMin=[]  IntegratorOutMax=[]  FilterOutMin=[]  FilterOutMax=[]  SumI1OutMin=[]  SumI1OutMax=[]  SumI2OutMin=[]  SumI2OutMax=[]  SumI3OutMin=[]  SumI3OutMax=[]  SumI4OutMin=[]  SumI4OutMax=[]  SumDOutMin=[]  SumDOutMax=[]  DifferentiatorOutMin=[]  DifferentiatorOutMax=[]  FilterDiffOutCoefMin=[]  FilterDiffOutCoefMax=[]  ReciprocalOutMin=[]  ReciprocalOutMax=[]  SumDenOutMin=[]  SumDenOutMax=[]  SumNumOutMin=[]  SumNumOutMax=[]  DivideOutMin=[]  DivideOutMax=[]  UdiffTsProdOutMin=[]  UdiffTsProdOutMax=[]  NTsProdOutMin=[]  NTsProdOutMax=[]  UintegralTsProdOutMin=[]  UintegralTsProdOutMax=[]  UngainTsProdOutMin=[]  UngainTsProdOutMax=[]  ClampingZeroOutDataTypeStr=Inherit: Inherit via back propagation  ClampingZeroOutMin=[]  ClampingZeroOutMax=[]  FilterDenConstantOutDataTypeStr=Inherit: Inherit via back propagation  FilterDenConstantOutMin=[]  FilterDenConstantOutMax=[]  PCopyOutDataTypeStr=Inherit: Inherit via back propagation  PCopyOutMin=[]  PCopyOutMax=[]  NCopyOutDataTypeStr=Inherit: Inherit via back propagation  NCopyOutMin=[]  NCopyOutMax=[]  IntegratorContinuousStateAttributes=''  IntegratorStateMustResolveToSignalObject=off  IntegratorRTWStateStorageClass=Auto  FilterContinuousStateAttributes=''  FilterStateMustResolveToSignalObject=off  FilterRTWStateStorageClass=Auto  ParallelPVariant=InternalParameters  IdealPVariant=Disabled  IVariant=InternalParameters  DVariant=Disabled  IntegratorVariant=Continuous  SatVariant=Disabled  AWVariant=Passthrough  PCopyVariant=Disabled  TRVariant=Disabled  FdbkBlocksVariant=Forward  IdealPFdbkVariant=Disabled  SatFdbkVariant=Disabled  DerivativeFilterVariant=Disabled  NVariant=Disabled  NCopyVariant=Disabled_SignalSpec  FilterICVariant=Disabled  IntegratorICVariant=InternalICs  ExternalResetVariant=Disabled  TRSumVariant=Passthrough  SumFdbkVariant=Disabled  SumVariant=Sum_PI  TsampFilterVariant=InternalTs  TsampNgainVariant=Passthrough  TsampIntegralVariant=Disabled_SignalSpec  ExternalSaturationOutDataTypeStr=Inherit: Same as second input
  Sum1 : Sum  Inputs=|-+
  Sum2 : Sum  Inputs=|+-
  Sum3 : Sum  Inputs=|++-
  Sum4 : Sum  Inputs=|+++
  abc to dq1 : spsabctodq0Lib/abc to dq0  Alignment=90 degrees behind phase A axis
  abc to dq3 : spsabctodq0Lib/abc to dq0  Alignment=90 degrees behind phase A axis
  wC : Gain  Gain=2*pi*50*15*10^-6
  Ild_ref : Outport
  Ilq_ref : Outport  Port=2
  wires:
  [V0d_W] -> Sum2/2, wC/1
  V0d_ref/1 -> Sum2/1
  Demux4/3 -> [V00_W]
  [V0q_W] -> Gain/1, Sum1/1
  Demux4/1 -> [V0d_W]
  V0_abc/1 -> abc to dq3/1
  Demux4/2 -> [V0q_W]
  abc to dq3/1 -> Demux4/1
  Sum2/1 -> PID Controller/1, DQ Errors/1
  PID Controller1/1 -> Sum4/2
  PID Controller/1 -> Sum3/2
  wC/1 -> Sum4/1
  Gain/1 -> Sum3/3
  V0q_ref/1 -> Sum1/2
  Sum1/1 -> PID Controller1/1, DQ Errors/2
  Sum3/1 -> Il ref/1, Ild_ref/1
  Sum4/1 -> Ilq_ref/1, Il ref/2
  Demux1/3 -> [Ig0_W]
  Demux1/1 -> [Igd_W]
  Ig_abc/1 -> abc to dq1/1
  Demux1/2 -> [Igq_W]
  abc to dq1/1 -> Demux1/1
  Wt/1 -> abc to dq1/2, abc to dq3/2
  [Igq_W] -> Sum4/3
  [Igd_W] -> Sum3/1

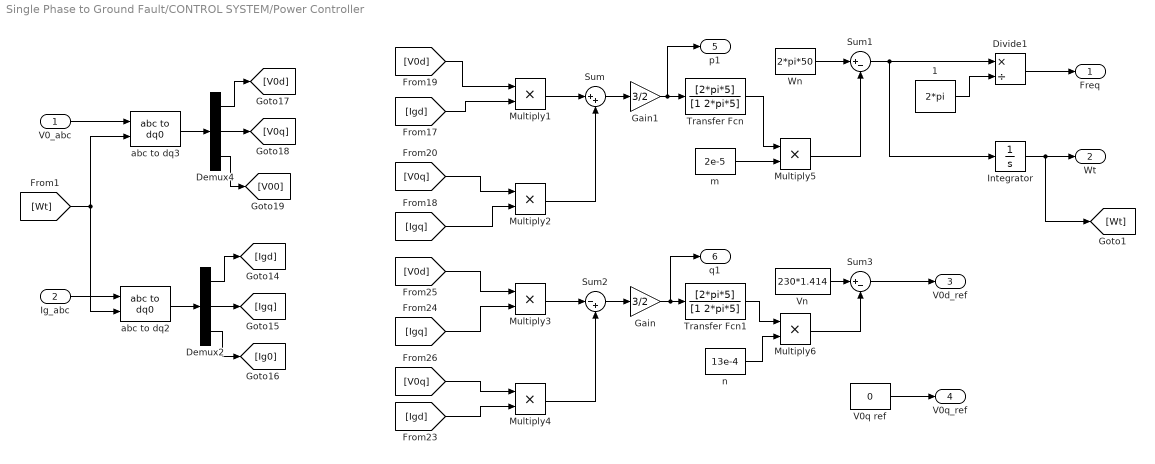
== system Single Phase to Ground Fault/CONTROL SYSTEM/Power Controller ==
  V0_abc : Inport
  Ig_abc : Inport  Port=2
  1 : Constant  Value=2*pi  SampleTime=Ts
  Demux2 : Demux  Outputs=3
  Demux4 : Demux  Outputs=3
  Divide1 : Product  Inputs=*/
  Gain : Gain  Gain=3/2
  Gain1 : Gain  Gain=3/2
  Integrator : Integrator
  Multiply{1..6} (6 alike) : Product  Inputs=**
  Sum : Sum  Inputs=|++
  Sum1 : Sum  Inputs=|+-
  Sum2 : Sum  Inputs=|-+
  Sum3 : Sum  Inputs=|+-
  Transfer Fcn : TransferFcn  Numerator=[2*pi*5]  Denominator=[1 2*pi*5]
  Transfer Fcn1 : TransferFcn  Numerator=[2*pi*5]  Denominator=[1 2*pi*5]
  V0q ref : Constant  Value=0  SampleTime=Ts
  Vn : Constant  Value=230*1.414  SampleTime=Ts
  Wn : Constant  Value=2*pi*50  SampleTime=Ts
  abc to dq2 : spsabctodq0Lib/abc to dq0  Alignment=90 degrees behind phase A axis
  abc to dq3 : spsabctodq0Lib/abc to dq0  Alignment=90 degrees behind phase A axis
  m : Constant  Value=2e-5  SampleTime=Ts
  n : Constant  Value=13e-4  SampleTime=Ts
  Freq : Outport
  Wt : Outport  Port=2
  V0d_ref : Outport  Port=3
  V0q_ref : Outport  Port=4
  p1 : Outport  Port=5
  q1 : Outport  Port=6
  wires:
  Transfer Fcn1/1 -> Multiply6/1
  Multiply5/1 -> Sum1/2
  Multiply6/1 -> Sum3/2
  Sum/1 -> Gain1/1
  Sum3/1 -> V0d_ref/1
  Sum2/1 -> Gain/1
  Gain1/1 -> p1/1, Transfer Fcn/1
  abc to dq3/1 -> Demux4/1
  V0_abc/1 -> abc to dq3/1
  Demux4/1 -> [V0d]
  Demux4/2 -> [V0q]
  Demux4/3 -> [V00]
  Demux2/2 -> [Igq]
  [Wt] -> abc to dq2/2, abc to dq3/2
  Ig_abc/1 -> abc to dq2/1
  Demux2/3 -> [Ig0]
  Demux2/1 -> [Igd]
  abc to dq2/1 -> Demux2/1
  [V0q] -> Multiply2/1
  [Igq] -> Multiply3/2
  Multiply3/1 -> Sum2/1
  [V0q] -> Multiply4/1
  [V0d] -> Multiply3/1
  [Igd] -> Multiply1/2
  [V0d] -> Multiply1/1
  Multiply2/1 -> Sum/2
  Multiply1/1 -> Sum/1
  [Igq] -> Multiply2/2
  [Igd] -> Multiply4/2
  Sum1/1 -> Integrator/1, Divide1/1
  Gain/1 -> q1/1, Transfer Fcn1/1
  m/1 -> Multiply5/2
  Multiply4/1 -> Sum2/2
  Wn/1 -> Sum1/1
  Transfer Fcn/1 -> Multiply5/1
  n/1 -> Multiply6/2
  Vn/1 -> Sum3/1
  V0q ref/1 -> V0q_ref/1
  1/1 -> Divide1/2
  Divide1/1 -> Freq/1
  Integrator/1 -> [Wt], Wt/1
